simulink model "Valve_Simulink"  (R2023a)
settings: Solver=VariableStepAuto  StartTime=0.0  StopTime=1  RelTol=1e-3
libraries: simulink x2
settings Model: Creator=xuluyu  LastModifiedBy=xuluyu

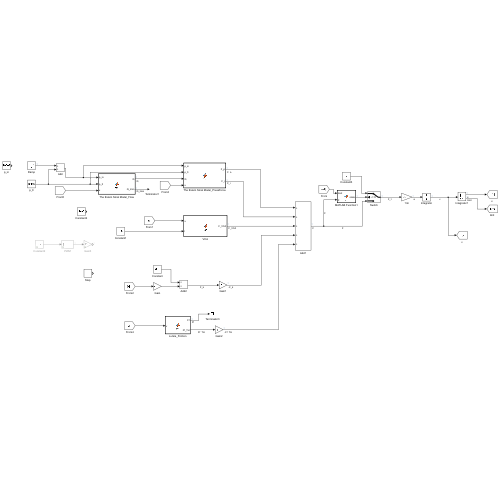
[thumbnail: Simulink's stored preview of the top-level diagram]
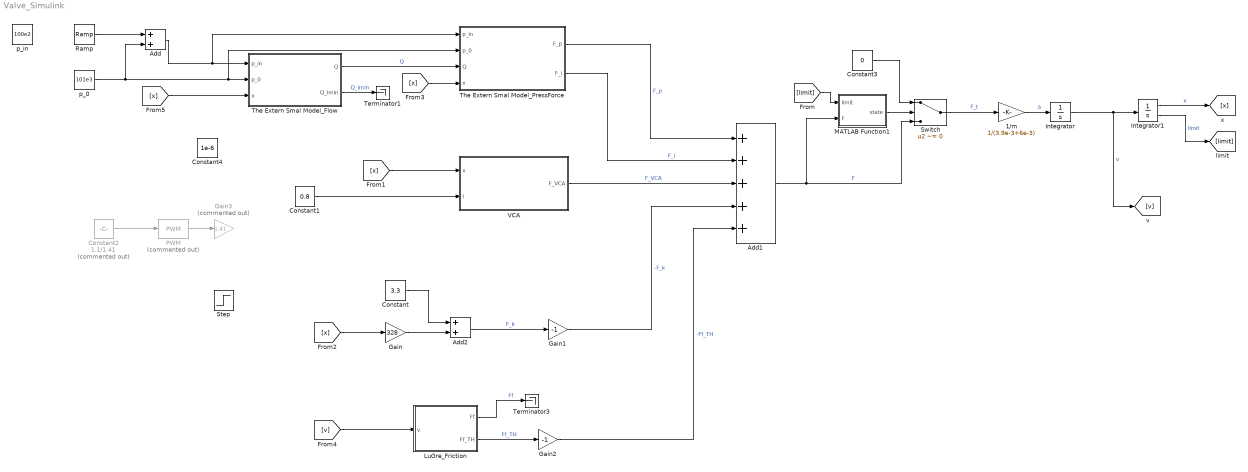
== system Valve_Simulink ==
  1/m : Gain  Gain=1/(3.9e-3+6e-3)
  Add : Sum
  Add1 : Sum  Inputs=+++++
  Add2 : Sum
  Constant : Constant  Value=3.3
  Constant1 : Constant  Value=0.8
  Constant2 : Constant  Commented=on  Value=1.1/1.41
  Constant3 : Constant  Value=0
  Constant4 : Constant  Value=1e-6
  Gain : Gain  Gain=328
  Gain1 : Gain  Gain=-1
  Gain2 : Gain  Gain=-1
  Gain3 : Gain  Commented=on  Gain=1.41
  Integrator : Integrator
  Integrator1 : Integrator  InitialCondition=1e-6  LimitOutput=on  UpperSaturationLimit=2e-3  LowerSaturationLimit=1e-6  ShowSaturationPort=on  ContinuousStateAttributes='x'
  LuGre_Friction : MATLAB Function  TreatAsAtomicUnit=on
  MATLAB Function1 : MATLAB Function  TreatAsAtomicUnit=on
  PWM : simulink/Discontinuities/PWM  Commented=on  DisableCoverage=on  Period=1/10e3  InitialDelay=0  DisallowZeroDutyCycle=off  RunAtFixedTimeIntervals=off  SampleTime=0.1
  Ramp : simulink/Sources/Ramp  slope=120e2  start=0.2  InitialOutput=0
  Step : Step  SampleTime=0
  Switch : Switch  Criteria=u2 ~= 0  SaturateOnIntegerOverflow=off  InputSameDT=off
  Terminator1 : Terminator
  Terminator3 : Terminator
  The Extern Smal Model_Flow : MATLAB Function  TreatAsAtomicUnit=on
  The Extern Smal Model_PressForce : MATLAB Function  TreatAsAtomicUnit=on
  VCA : MATLAB Function  TreatAsAtomicUnit=on
  p_0 : Constant  Value=101e3
  p_in : Constant  Value=100e2
  wires:
  Integrator/1 -> [v], Integrator1/1  "v"
  Add2/1 -> Gain1/1  "F_k"
  1/m/1 -> Integrator/1  "a"
  LuGre_Friction/2(Ff_TH) -> Gain2/1  "Ff_TH"
  LuGre_Friction/1(Ff) -> Terminator3/1  "Ff"
  Switch/1 -> 1/m/1  "F_t"
  Constant3/1 -> Switch/1
  MATLAB Function1/1(state) -> Switch/2
  Constant/1 -> Add2/1
  Add1/1 -> Switch/3, MATLAB Function1/2(F)  "F"
  Integrator1/1 -> [x]  "x"
  Integrator1/2 -> [limit]  "limit"
  [limit] -> MATLAB Function1/1(limit)
  The Extern Smal Model_Flow/1(Q) -> The Extern Smal Model_PressForce/3(Q)  "Q"
  p_0/1 -> Add/2, The Extern Smal Model_PressForce/2(p_0), The Extern Smal Model_Flow/2(p_0)
  Add/1 -> The Extern Smal Model_PressForce/1(p_in), The Extern Smal Model_Flow/1(p_in)
  The Extern Smal Model_Flow/2(Q_lmin) -> Terminator1/1  "Q_lmin"
  [x] -> Gain/1
  [v] -> LuGre_Friction/1(v)
  The Extern Smal Model_PressForce/1(F_p) -> Add1/1  "F_p"
  The Extern Smal Model_PressForce/2(F_i) -> Add1/2  "F_i"
  VCA/1(F_VCA) -> Add1/3  "F_VCA"
  Gain1/1 -> Add1/4  "-F_k"
  Gain/1 -> Add2/2
  Ramp/1 -> Add/1
  Gain2/1 -> Add1/5  "-Ff_TH"
  PWM/1 -> Gain3/1
  Constant2/1 -> PWM/1
  Constant1/1 -> VCA/2(I)
  [x] -> VCA/1(x)
  [x] -> The Extern Smal Model_PressForce/4(x)
  [x] -> The Extern Smal Model_Flow/3(x)

== matlab function Valve_Simulink/The Extern Smal Model_Flow ==
  data: p_in input; p_0 input; x input; Q output; Q_lmin output
function [Q,Q_lmin] = fcn(p_in,p_0,x)
% The Extended Smal Model
% 拓展的smal模型，包括流量模型
% 阀座和膜片的几何参数
r_vi= 5e-3;%阀内进气腔半径，m
r_in = 5e-3;%阀外进气口半径，m
r_c = 6e-3;%阀内进气腔末端半径，m
r_m = 5e-3;%膜片半径，m
r_ex = 5e-3;%阀外出气口半径，m
% 流量模型-Flow Medel
% p_0 = 101e3;%阀外出口压力，Pa,(默认为标准大气压)
% p_in = 10e2+p_0;%阀外进气口压力,Pa
zeta_in = 1-(r_vi/r_in)^4;%阀进气口的压力损失因子，1
zeta_ex = 1-(r_ex/r_c)^4;%阀出气口的压力损失因子，1
% x_det_max = 2e-3;%线圈最大位移，m
% x_det = 1e-4:1e-4:(x_det_max);%线圈位移，即阀口位移，m
yr = x/(2*r_vi);%
zeta_yr = -6.1*exp(-4.13*yr)+0.497*(yr.^(-1.29))+1;%压力调整系数 
mu_air = 1.7894e-5;%空气粘度系数，Pa*s
rho_air = 1.248;%空气密度，kg/m^3
g1 = pi/(12*mu_air)*(r_c+r_in)/(r_c-r_in);
g2 = rho_air/2*g1*(1/(pi*r_in^2))^2;
g3 = rho_air/2*g1*(1/(pi*r_ex^2))^2;
g4 = rho_air/2*g1*(1/(2*pi*r_in))^2;
Q = (-1+sqrt(1+4*((zeta_yr+zeta_in-1)*g2*x^3+zeta_ex*g3*x^3+g4*x)*g1*x^3*(p_in-p_0)))...
        /(2*((zeta_yr+zeta_in-1)*g2*x^3+zeta_ex*g3*x^3+g4*x));%m^3/s
% Q = (-1+siqrt(1+4*((zeta_yr+zeta_in-1)*g2.*x.^3+zeta_ex*g3*x.^3+g4.*x).*g1.*x.^3*(p_in-p_0)))...
%     ./2*((zeta_yr+zeta_in-1)*g2.*x.^3+zeta_ex*g3.*x.^3+g4.*x);
Q_lmin = Q*1e3*60;
end

== matlab function Valve_Simulink/VCA ==
  data: x input; F_VCA output; I input
function F_VCA  = fcn(x, I)
% VCA
% 音圈电磁力模型
% Pg-气隙磁导
% 默认音圈的永磁铁为圆柱形式
mu_0 = pi*4e-7;%磁导率，N*A^-2
r1 = 12e-3;%极片半径，m
r2 = 20e-3;%外壳半径，m
h = 10e-3;%极片高度，m
%Ag = (r2-r1)*h;%气隙磁路横截面，m^2
Ag = 2*pi*(r2+r1)*h;%气隙面积，m^2
Lg = 2*pi*(r1+r2)/2;%气隙长度，m
Pg = mu_0*Ag/Lg;%气隙磁导,H/m
%  气隙外总泄露磁导-Ptl
Dp = r1*2;%极片直径，m
Dy = r2*2;%扼片直径，m
Dm = 10e-3*2;%磁铁直径，m
Lm = 10e-3;%磁铁长度，m
Pf1 = 0.264*pi*mu_0*(Dp+Lg);
Pf2 = mu_0*(Dp+Lg)*log(1+Dp/Lg);
Pf3 = mu_0*(Dp+Lg)*log(1+(Dp-Dm)/Lg);
Pi = pi*mu_0*Lm*(Dm+Dy)/(4*(Dy-Dm));
Pl = pi*mu_0*sqrt(Dm*Lm/2);
P_ex = max(Pi,Pl);
Ptl = Pf1+Pf2+Pf3+P_ex;%气隙外总泄露磁导
% 磁导泄露系数-sigma
Pt = Pg+Ptl;%电路的总磁导
sigma = Pt/Pg;%磁导泄露系数
% 实际磁导-Pc
Am = 2*pi*(Dm/2)^2+2*pi*(Dm/2)*Lm;%磁铁面积，m^2
Pc = mu_0*(Ag*Lm/(Am*Lg))*sigma;
% 工作点的磁通密度-Bd
Br = 20;%最大磁通密度，H，不确定
mu_rec = 1*mu_0;%相对磁导率，不确定
Bd = Br/(1+mu_rec/Pc);
% 气隙的磁通密度-Bg
Bg = Am*Bd/(Ag*sigma);%气隙的磁通密度
% 气隙外磁通密度的归一化函数-Bnorm
ks = 20;%优化参数，针对不同的音圈需要调整
Bnorm = Lg/(ks*pi*x+Lg);
% 气隙上下的磁通密度-Ba,Bb
Ba = Bg*Bnorm;
Bb = Ba;
% 电磁力系数-Bl
% x_det_max = 9e-3;%线圈最大位移，m
% x_init = 0e-3;%线圈初始位移，m
xi = 5e-3;%内部线圈长度，m，小于Lm
xg = h/2;%气隙线圈长度，m
xo = 10e-4;%外部线圈长度，m
Number_Of_CoilTurns = 10e3;% 线圈匝数
% length_of_coil = 2e-3;% 线圈宽度，m
li = (xi-x)*2*pi*r1;
lg = xg*2*pi*r1;
lo = (xo+x)*2*pi*r1;
B_li = Bg*Lg*log(Lg+pi*ks*li)/(ks*pi)-Bg*Lg*log(Lg+pi*ks*0)/(ks*pi);
B_lg = Bg*lg;
B_lo = Bg*Lg*log(Lg+pi*ks*lo)/(ks*pi)-Bg*Lg*log(Lg+pi*ks*0)/(ks*pi);
B_t = (B_li+B_lg+B_lo)*Number_Of_CoilTurns;
% 电磁力-F
% I = 1;%线圈电流，A
F_VCA = B_t * I;
end

== matlab function Valve_Simulink/The Extern Smal Model_PressForce ==
  data: p_in input; p_0 input; Q input; x input; F_p output; F_i output
function [F_p,F_i] = fcn(p_in,p_0,Q,x)
% The Extended Smal Model
% 拓展的smal模型，包括流量模型、压力模型
% 阀座和膜片的几何参数
r_vi= 5e-3;%阀内进气腔半径，m
r_in = 5e-3;%阀外进气口半径，m
r_c = 6e-3;%阀内进气腔末端半径，m
r_m = 5e-3;%膜片半径，m
r_ex = 5e-3;%阀外出气口半径，m
% 流量模型-Flow Medel
zeta_in = 1-(r_vi/r_in)^4;%阀进气口的压力损失因子，1
zeta_ex = 1-(r_ex/r_c)^4;%阀出气口的压力损失因子，1
% x_det_max = 5e-3;%线圈最大位移，m
yr = x/(2*r_vi);%
zeta_yr = -6.1*exp(-4.13*yr)+0.497*(yr.^(-1.29))+1;%压力调整系数 
mu_air = 1.7894e-5;%空气粘度系数，Pa*s
rho_air = 1.248;%空气密度，kg/m^3
% 拓展的smal压力模型
p_vi = p_in - zeta_in*(rho_air/2).*(Q./(pi*r_vi^2)).^2;%阀内进气腔压力，Pa
p_c = p_0 + zeta_ex*(rho_air/2).*(Q./(pi*r_ex^2)).^2;%阀内进气腔末端压力，Pa
% 压力分布模型
n_yr = -29*exp(-77.2*yr)+27.8*exp(-17.5*yr);%压力分布指数
p1 = p_vi+rho_air/2*(Q/(pi*(r_vi)^2)).^2;%膜片中心压力
p2 = p1-rho_air/2*(Q./(2*pi*r_vi*x)).^2;%进气腔与膜片的交界处的压力
% 压力模型-Press Force Model
% a1 = pi*r_vi^2/2;
% a2 = pi*r_vi^2/2+pi*(pi*r_c^3+2*r_vi^3-3*r_c*r_vi^2)/(3*(r_c-r_vi));
a1 = n_yr./(n_yr+2)*(pi*r_vi^2);
a2 = 2./(n_yr+2)*pi*r_vi^2+pi*(pi*r_c^3+2*r_in^3-3*r_c*r_in^2)/(3*(r_c-r_in));
a3 = -1*pi*(pi*r_c^3+2*r_vi^3-3*r_c*r_vi^2)/(3*(r_c-r_vi))+pi*r_m^2-pi*r_vi^2;
a4 = pi*r_m^2;
F_p = a1*p1+a2*p2+a3*p_c-a4*p_0;% 膜片所受压力
F_i = 2*rho_air*Q.^2/(pi*r_in^2);% 流量导致的惯性力
end

== matlab function Valve_Simulink/LuGre_Friction ==
  data: v input; Ff output; Ff_TH output
function [Ff,Ff_TH] = fcn(v)
% LuGre_Friction
% LuGre摩擦力模型
% Columb-库伦摩擦-Fc
mu_c = 0.10;%动摩擦系数
Fn = 2;%法向力,N
Fc = mu_c*Fn;%库伦摩擦,N
% Viscous-粘性摩擦-Fv
% deta_v = 17.9e-6;%粘性系数，N*m^2/s
deta_v = 8e-4;%粘性系数，N*m^2/s 8e-1
Fv = deta_v*v;
% brk-临界摩擦-Fbrk
mu_b = 0.15;%临界(静)摩擦系数
Fbrk = mu_b*Fn;%临界摩擦,N
% Stribeck-斯特里贝克摩擦-Fs
cv = 100;
Fs = (Fbrk-Fc)*exp(-1*cv*abs(v))*sign(v);
% 总摩擦力-Ff
Ff = Fc+Fv+Fs;
% 总摩擦力-Ff
v_TH = 1e-4;% 速度阈值，m/s
if(abs(v)<v_TH)
    Ff_TH = abs(v)*sign(v)*(Fc+(Fbrk-Fc)*exp(-1*cv*v_TH))/v_TH;
else
    Ff_TH = Fc+((Fbrk-Fc)*exp(-1*cv*abs(v))*sign(v))+Fv;
end
end

== matlab function Valve_Simulink/MATLAB Function1 ==
  data: limit input; state output; F input
function state = fcn(limit,F)
if(limit==1 && F>0)
    state = 1;
elseif(limit==-1 && F<0)
    state = -1;
else
    state = 0;
end
